simulink model "TRAINING_MATLAB_II_ex2_6a"  (R2019b)
settings: Solver=ode3  StartTime=0.0  StopTime=100.0  FixedStep=0.01  RelTol=1e-3
undefined symbols (not defined in the file): DiscIntNeverNeededParam
libraries: simulink x2
settings Model: EnablePacing=on  Creator=Laura  LastModifiedBy=Pablo

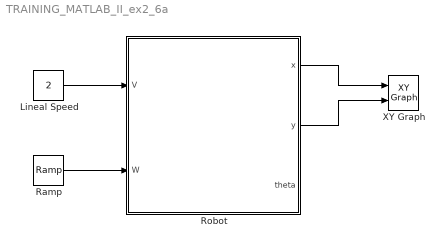
== system TRAINING_MATLAB_II_ex2_6a ==
  Lineal Speed : Constant  Value=2
  "Ramp " : simulink/Sources/Ramp  slope=1  start=0  InitialOutput=0
  "Robot " : Subsystem
  XY Graph : simulink/Sinks/XY Graph  xmin=-10  xmax=10  ymin=-10  ymax=10  st=-1
  wires:
  Lineal Speed/1 -> "Robot "/1(V)
  "Ramp "/1 -> "Robot "/2(W)
  "Robot "/1(x) -> XY Graph/1
  "Robot "/2(y) -> XY Graph/2

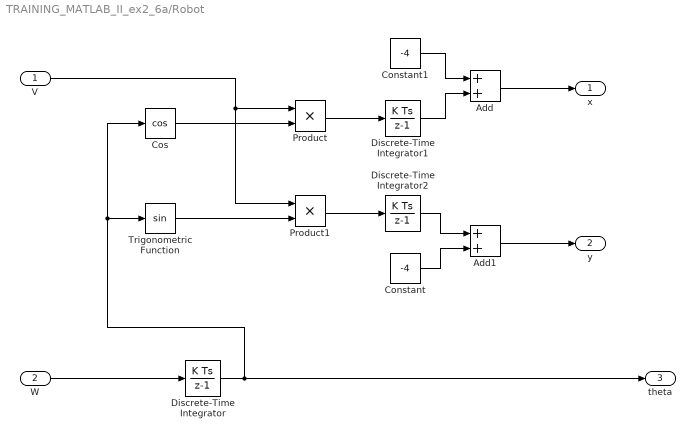
== system TRAINING_MATLAB_II_ex2_6a/Robot  ==
  V : Inport
  W : Inport  Port=2
  Add : Sum
  Add1 : Sum
  Constant : Constant  Value=-4
  Constant1 : Constant  Value=-4
  Cos : Trigonometry  Operator=cos
  Discrete-Time Integrator : DiscreteIntegrator  SampleTime=-1  ICPrevOutput=DiscIntNeverNeededParam  ICPrevScaledInput=DiscIntNeverNeededParam
  Discrete-Time Integrator1 : DiscreteIntegrator  SampleTime=-1  ICPrevOutput=DiscIntNeverNeededParam  ICPrevScaledInput=DiscIntNeverNeededParam
  Discrete-Time Integrator2 : DiscreteIntegrator  SampleTime=-1  ICPrevOutput=DiscIntNeverNeededParam  ICPrevScaledInput=DiscIntNeverNeededParam
  Product : Product
  Product1 : Product
  Trigonometric Function : Trigonometry
  x : Outport
  y : Outport  Port=2
  theta : Outport  Port=3
  wires:
  Discrete-Time Integrator/1 -> theta/1, Cos/1, Trigonometric Function/1
  V/1 -> Product1/1, Product/1
  W/1 -> Discrete-Time Integrator/1
  Cos/1 -> Product/2
  Trigonometric Function/1 -> Product1/2
  Constant/1 -> Add1/2
  Constant1/1 -> Add/1
  Product/1 -> Discrete-Time Integrator1/1
  Product1/1 -> Discrete-Time Integrator2/1
  Discrete-Time Integrator2/1 -> Add1/1
  Add1/1 -> y/1
  Discrete-Time Integrator1/1 -> Add/2
  Add/1 -> x/1
